simulink subsystem "RADAR_MIPI_I2C"  (R2022b)
settings: Solver=VariableStepAuto  StartTime=0.0  StopTime=10.0  RelTol=1e-3
libraries: simulink x2, hdlsllib x1
Description:
  | Copyright (c) 2023, Alexei Evsenin, evsenin@gmail.com
settings Model: Creator=evsenin  LastModifiedBy=evsenin
settings ModelReferenceCC: EnableRefExpFcnMdlSchedulingChecks=on

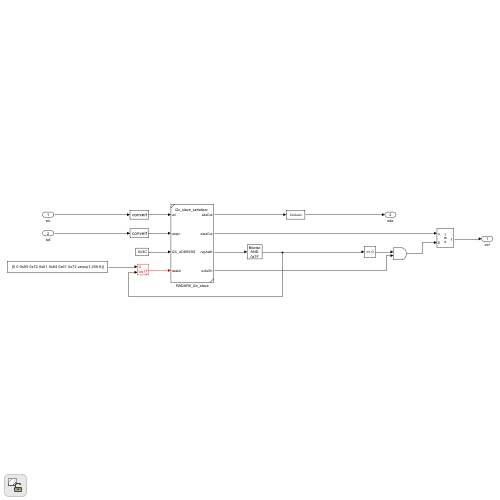
[thumbnail: Simulink's stored preview of the top-level diagram]
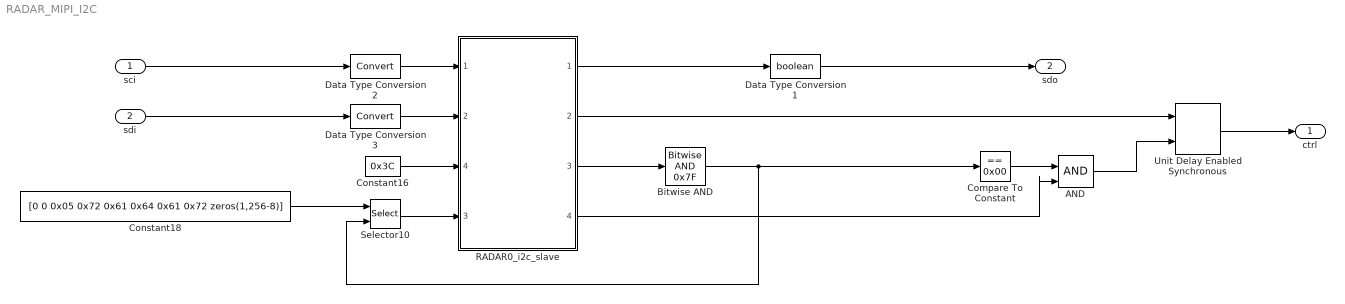
== system RADAR_MIPI_I2C ==
  sci : Inport
  sdi : Inport  Port=2
  AND : Logic  IconShape=distinctive  AllPortsSameDT=off  OutDataTypeStr=boolean
  Bitwise AND : simulink/Logic and Bit Operations/Bitwise Operator  logicop=AND  UseBitMask=on  BitMask=0x7F  BitMaskRealWorld=Stored Integer
  Compare To Constant : simulink/Logic and Bit Operations/Compare To Constant  relop===  const=0x00  OutDataTypeStr=boolean
  Constant16 : Constant  Value=0x3C  OutDataTypeStr=fixdt(0,7,0)  SampleTime=-1
  Constant18 : Constant  Value=[0 0 0x05 0x72 0x61 0x64 0x61 0x72 zeros(1,256-8)]  OutDataTypeStr=uint8  SampleTime=-1
  Data Type Conversion1 : DataTypeConversion  OutDataTypeStr=boolean  SaturateOnIntegerOverflow=off  RndMeth=Floor
  Data Type Conversion2 : DataTypeConversion  SaturateOnIntegerOverflow=off  RndMeth=Floor
  Data Type Conversion3 : DataTypeConversion  SaturateOnIntegerOverflow=off  RndMeth=Floor
  RADAR0_i2c_slave : Subsystem  ReferencedSubsystem=i2c_slave_serializer
      settings: PortSchema="{\"entries\":[{\"content\":{\"sides\":[{\"content\":{\"connectorIds\":[\"In1\",\"In2\",\"In4\",\"In3\"]},\"type\":\"ConnectorPlacement.EquallySpacedRectSide\",\"uuid\":\"5cabedeb-c807-4889-8ba0-5ab9031a84ba\"},{\"content\":{\"connectorIds\":[\"Out1\",\"Out2\",\"Out3\",\"Out4\"],\"side\":\"RIGHT\"},\"type\":\"ConnectorPlacement.EquallySpacedRectSide\",\"uuid\":\"ca7acdc8-82b2-4681-aa13-89f67544921e\"},{\"content\":{\"connectorIds\":[],\"side\":\"TOP\"},\"type\":\"ConnectorPlacement.EquallySpacedRectSide\",\"uuid\":\"8b24d124-fa07-455d-a189-f258fbea822f\"}]},\"type\":\"ConnectorPlacement.EquallySpacedConnector\",\"uuid\":\"6802f4c9-cf5e-4fdc-ad1f-26d27f7bb24e\"}],\"packageUris\":[\"http://schema.mathworks.com/mf0/Connector/R2020b\"],\"version\":\"1.0\"}"
  Selector10 : Selector  IndexMode=Zero-based  IndexOptions=Index vector (port)  Indices=0  OutputSizes=1
  Unit Delay Enabled Synchronous : hdlsllib/Discrete/Unit Delay Enabled Synchronous  InitialCondition=0xFF  SampleTime=-1
  ctrl : Outport
  sdo : Outport  Port=2
  wires:
  AND/1 -> Unit Delay Enabled Synchronous/2
  Constant16/1 -> RADAR0_i2c_slave/4
  RADAR0_i2c_slave/1 -> Data Type Conversion1/1
  Data Type Conversion2/1 -> RADAR0_i2c_slave/1
  Bitwise AND/1 -> Selector10/2, Compare To Constant/1
  Data Type Conversion3/1 -> RADAR0_i2c_slave/2
  sci/1 -> Data Type Conversion2/1
  RADAR0_i2c_slave/4 -> AND/2
  sdi/1 -> Data Type Conversion3/1
  Selector10/1 -> RADAR0_i2c_slave/3
  RADAR0_i2c_slave/2 -> Unit Delay Enabled Synchronous/1
  Compare To Constant/1 -> AND/1
  Constant18/1 -> Selector10/1
  RADAR0_i2c_slave/3 -> Bitwise AND/1
  Unit Delay Enabled Synchronous/1 -> ctrl/1
  Data Type Conversion1/1 -> sdo/1
